simulink model "V_select"  (R2025b)
settings: Solver=ode4  StartTime=0.0  StopTime=10.0  FixedStep=0.1  RelTol=1e-3
libraries: simulink x2, dspstat3 x2
settings Model: Creator=Pragati-TRN0433  LastModifiedBy=Pragati-TRN0433

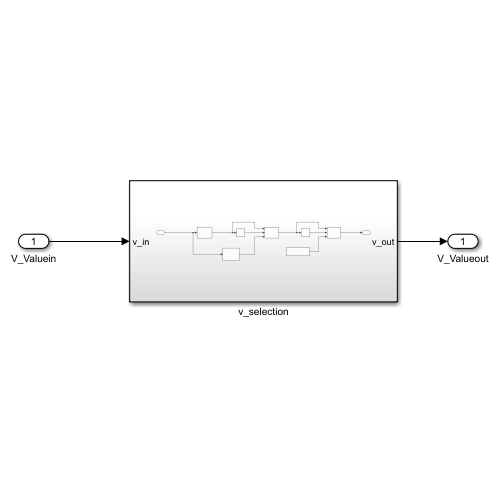
[thumbnail: Simulink's stored preview of the top-level diagram]
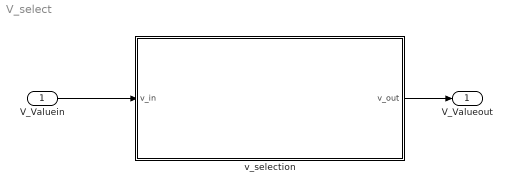
== system V_select ==
  V_Valuein : Inport  OutDataTypeStr=single
  v_selection : Subsystem
  V_Valueout : Outport  OutDataTypeStr=single
  wires:
  V_Valuein/1 -> v_selection/1(v_in)
  v_selection/1(v_out) -> V_Valueout/1

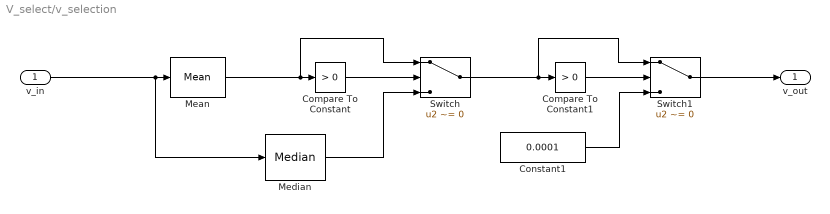
== system V_select/v_selection ==
  v_in : Inport
  Compare To Constant : simulink/Logic and Bit Operations/Compare To Constant  relop=>  const=0  OutDataTypeStr=boolean
  Compare To Constant1 : simulink/Logic and Bit Operations/Compare To Constant  relop=>  const=0  OutDataTypeStr=boolean
  Constant1 : Constant  Value=0.0001  OutDataTypeStr=single
  Mean : dspstat3/Mean  run=off  InputProcessing=Columns as channels (frame based)  reset_popup=None  directionMode=Each column  dimension=1  roiEnable=off  roiType=Rectangles  roiPortion=Entire ROI  roiOutput=Individual statistics for each ROI  roiFlag=off  roundingMode=Floor  overflowMode=off  outputDataTypeStr=Inherit: Same as accumulator  outputMin=[]  outputMax=[]  outputLastDataTypeStr=Inherit: Same as accumulator
  Median : dspstat3/Median  sortAlg=Quick sort  directionMode=Each column  dimension=1  roundingMode=Floor  overflowMode=off  accumDataTypeStr=Inherit: Same as product output  accumLastDataTypeStr=Inherit: Same as product output  outputDataTypeStr=Inherit: Same as accumulator  outputMin=[]  outputMax=[]  outputLastDataTypeStr=Inherit: Same as accumulator
      settings: allowOverrides=off
  Switch : Switch  Criteria=u2 ~= 0  SaturateOnIntegerOverflow=off  InputSameDT=off
  Switch1 : Switch  Criteria=u2 ~= 0  SaturateOnIntegerOverflow=off  InputSameDT=off
  v_out : Outport
  wires:
  v_in/1 -> Median/1, Mean/1
  Mean/1 -> Switch/1, Compare To Constant/1
  Median/1 -> Switch/3
  Compare To Constant/1 -> Switch/2
  Switch/1 -> Switch1/1, Compare To Constant1/1
  Compare To Constant1/1 -> Switch1/2
  Switch1/1 -> v_out/1
  Constant1/1 -> Switch1/3
